simulink model "Op_Space_Inv_Dyn"  (R2020b)
settings: Solver=VariableStepAuto  StartTime=0.0  StopTime=tk(end)-tk(1)  RelTol=1e-3
values from neighbouring files (symbols this model uses):
  B = myRobot.B_Lagrangian    [hw10_main.m]
  C = myRobot.C_Lagrangian    [hw10_main.m]
  dJa = dJa(1:3,:)    [hw10_main.m]
  F = myRobot.F    [hw10_main.m]
  G = myRobot.G_Lagrangian    [hw10_main.m]
  Ja = Ja(1:3,:)    [hw10_main.m]
  Ja_inv = inv(Ja)    [hw10_main.m]
  Kd = diag([1 1 1]).*5    [hw10_main.m]
  Kp = diag([1 1 1]).*100    [hw10_main.m]
  Ts = 0.001    [hw10_main.m]
settings Model: Creator=nicol  LastModifiedBy=nicol

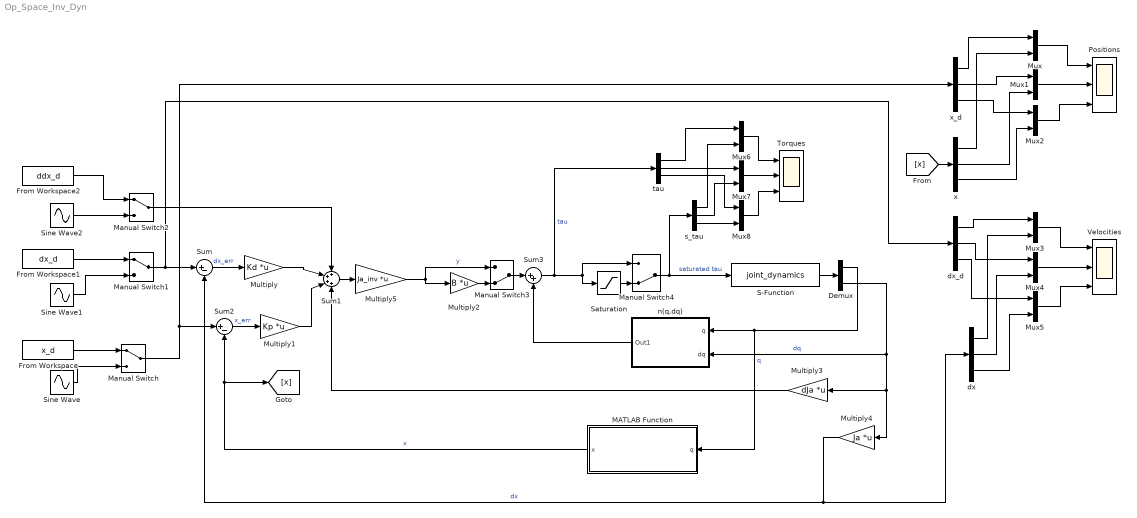
== system Op_Space_Inv_Dyn ==
  Demux : Demux  Outputs=2
  From Workspace : FromWorkspace  VariableName=x_d  SampleTime=Ts
  From Workspace1 : FromWorkspace  VariableName=dx_d  SampleTime=Ts
  From Workspace2 : FromWorkspace  VariableName=ddx_d  SampleTime=Ts
  MATLAB Function : MATLAB Function  TreatAsAtomicUnit=on
  Manual Switch : ManualSwitch
  Manual Switch1 : ManualSwitch
  Manual Switch2 : ManualSwitch
  Manual Switch3 : ManualSwitch  CurrentSetting=0
  Manual Switch4 : ManualSwitch  CurrentSetting=0
  Multiply : Gain  Gain=Kd  Multiplication=Matrix(K*u)
  Multiply1 : Gain  Gain=Kp  Multiplication=Matrix(K*u)
  Multiply2 : Gain  Gain=B  Multiplication=Matrix(K*u)
  Multiply3 : Gain  Gain=dJa  Multiplication=Matrix(K*u)
  Multiply4 : Gain  Gain=Ja  Multiplication=Matrix(K*u)
  Multiply5 : Gain  Gain=Ja_inv  Multiplication=Matrix(K*u)
  Mux{,1..8} (9 alike) : Mux  Inputs=2
  Positions : Scope  NumInputPorts=3
  S-Function : S-Function  FunctionName=joint_dynamics  Parameters=myRobot  SFunctionDeploymentMode=off  EnableBusSupport=off
  Saturation : Saturate  UpperLimit=50  LowerLimit=-50
  Sine Wave : Sin  Amplitude=0.1  SampleTime=0  VectorParams1D=off
  Sine Wave1 : Sin  Amplitude=0.1  SampleTime=0  VectorParams1D=off
  Sine Wave2 : Sin  Amplitude=0.1  SampleTime=0  VectorParams1D=off
  Sum : Sum  Inputs=|+-
  Sum1 : Sum  Inputs=++++
  Sum2 : Sum  Inputs=|+-
  Sum3 : Sum  Inputs=|++
  Torques : Scope  NumInputPorts=3
  Velocities : Scope  NumInputPorts=3
  dx : Demux  Outputs=3
  dx_d : Demux  Outputs=3
  n(q,dq) : Subsystem
  s_tau : Demux  Outputs=3
  tau : Demux  Outputs=3
  x : Demux  Outputs=3
  x_d : Demux  Outputs=3
  wires:
  From Workspace1/1 -> Manual Switch1/1
  Sum/1 -> Multiply/1  "dx_err"
  Multiply/1 -> Sum1/2
  From Workspace/1 -> Manual Switch/1
  Sum2/1 -> Multiply1/1  "x_err"
  Multiply1/1 -> Sum1/3
  Multiply2/1 -> Manual Switch3/2
  Sum3/1 -> Manual Switch4/1, Saturation/1, tau/1  "tau"
  S-Function/1 -> Demux/1
  Demux/1 -> n(q,dq)/1(q), MATLAB Function/1(q)  "q"
  Demux/2 -> n(q,dq)/2(dq), Multiply4/1, Multiply3/1  "dq"
  n(q,dq)/1(Out1) -> Sum3/2
  From Workspace2/1 -> Manual Switch2/1
  x/2 -> Mux1/2
  x/3 -> Mux2/2
  x/1 -> Mux/2
  Sine Wave/1 -> Manual Switch/2
  Sine Wave1/1 -> Manual Switch1/2
  Sine Wave2/1 -> Manual Switch2/2
  Manual Switch2/1 -> Sum1/1
  Manual Switch1/1 -> Sum/1, dx_d/1
  x_d/1 -> Mux/1
  x_d/2 -> Mux1/1
  x_d/3 -> Mux2/1
  Mux/1 -> Positions/1
  Mux1/1 -> Positions/2
  Mux2/1 -> Positions/3
  Mux3/1 -> Velocities/1
  dx_d/3 -> Mux5/1
  Mux4/1 -> Velocities/2
  Mux5/1 -> Velocities/3
  dx_d/2 -> Mux4/1
  dx/1 -> Mux3/2
  dx_d/1 -> Mux3/1
  dx/3 -> Mux5/2
  Manual Switch/1 -> Sum2/1, x_d/1
  dx/2 -> Mux4/2
  tau/2 -> Mux7/1
  tau/1 -> Mux6/1
  s_tau/1 -> Mux6/2
  s_tau/2 -> Mux7/2
  tau/3 -> Mux8/1
  s_tau/3 -> Mux8/2
  Mux6/1 -> Torques/1
  Mux7/1 -> Torques/2
  Mux8/1 -> Torques/3
  Manual Switch3/1 -> Sum3/1
  MATLAB Function/1(x) -> [x], Sum2/2  "x"
  Multiply3/1 -> Sum1/4
  Multiply4/1 -> Sum/2, dx/1  "dx"
  Sum1/1 -> Multiply5/1
  Multiply5/1 -> Manual Switch3/1, Multiply2/1  "y"
  [x] -> x/1
  Manual Switch4/1 -> S-Function/1, s_tau/1  "saturated tau"
  Saturation/1 -> Manual Switch4/2

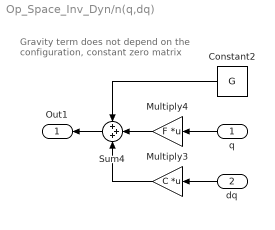
== system Op_Space_Inv_Dyn/n(q,dq) ==
  note: Gravity term does not depend on the
      |  configuration, constant zero matrix
  q : Inport
  dq : Inport  Port=2
  Constant2 : Constant  Value=G  VectorParams1D=off
  Multiply3 : Gain  Gain=C  Multiplication=Matrix(K*u)
  Multiply4 : Gain  Gain=F  Multiplication=Matrix(K*u)
  Sum4 : Sum  Inputs=+++
  Out1 : Outport
  wires:
  Sum4/1 -> Out1/1
  Multiply3/1 -> Sum4/3
  Multiply4/1 -> Sum4/2
  Constant2/1 -> Sum4/1
  q/1 -> Multiply4/1
  dq/1 -> Multiply3/1

== matlab function Op_Space_Inv_Dyn/MATLAB Function ==
  data: q input size=3; x output size=3
function x = directKinematics(q)
x=[ q(1) + 1/5;
    q(3) + 1/5;
    q(2) + 1251/5000];
end
